simulink model "strain"  (R2024b)
settings: Solver=FixedStepAuto  StartTime=0.0  StopTime=inf  RelTol=1e-3  EnableMultiTasking=on
libraries: fl_lib x5, nesl_utility x4, stm32f4xxblockslib x2, ee_lib x2
settings Model: STM32="{\"AnalogInput\":[{\"ID\":\"untitled1:2\"},{\"ID\":\"strain:206\"}],\"DigitalPortRead\":{\"ID\":\"strain:210\"}}"  Creator=Lenovo  LastModifiedBy=Lenovo
settings OptimizationCC: BlockReduction=off  DefaultParameterBehavior=Inlined  BufferReuse=off  EnhancedBackFolding=on  PassReuseOutputArgsAs=Individual arguments  ZeroExternalMemoryAtStartup=off  ZeroInternalMemoryAtStartup=off  MaxStackSize=512  OptimizeBlockOrder=speed  DifferentSizesBufferReuse=on  EfficientTunableParamExpr=on
settings DebuggingCC: ParameterTunabilityLossMsg=error
settings HardwareCC: ProdBitPerPointer=32  ProdBitPerSizeT=32  ProdBitPerPtrDiffT=32  ProdLargestAtomicInteger=Long  ProdLargestAtomicFloat=Double  ProdWordSize=32  ProdLongLongMode=on  ProdHWDeviceType=ARM Compatible->ARM Cortex-M
settings SFSimCC: MATLABDynamicMemAlloc=off
settings RTWCC: Description=Embedded Coder  SystemTargetFile=ert.tlc  HardwareBoard=STM32G4xx Based  TemplateMakefile=ert_default_tmf  Toolchain=GNU Tools for ARM Embedded Processors
settings CodeAppCC: ForceParamTrailComments=on  IgnoreCustomStorageClasses=off  OperatorAnnotations=on  SimulinkDataObjDesc=on  SFDataObjDesc=on  InsertBlockDesc=on
settings ERTTargetCC: TargetLangStandard=C99 (ISO)  CodeReplacementLibrary=ARM Cortex-M  ExtModeTransport=3  ExtModeStaticAlloc=on  ExtModeStaticAllocSize=2048  ExtModeMexFile=ext_xcp  ExtModeIntrfLevel=Level2 - Open

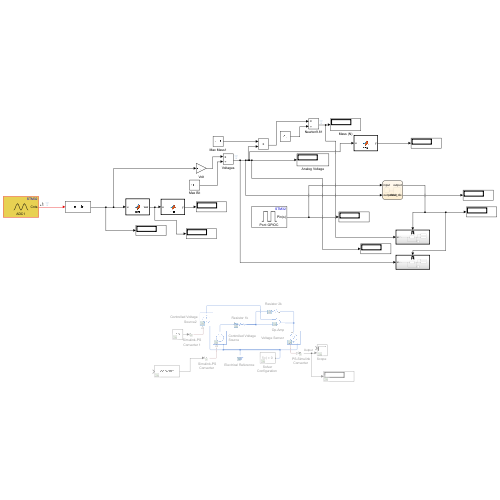
[thumbnail: Simulink's stored preview of the top-level diagram]
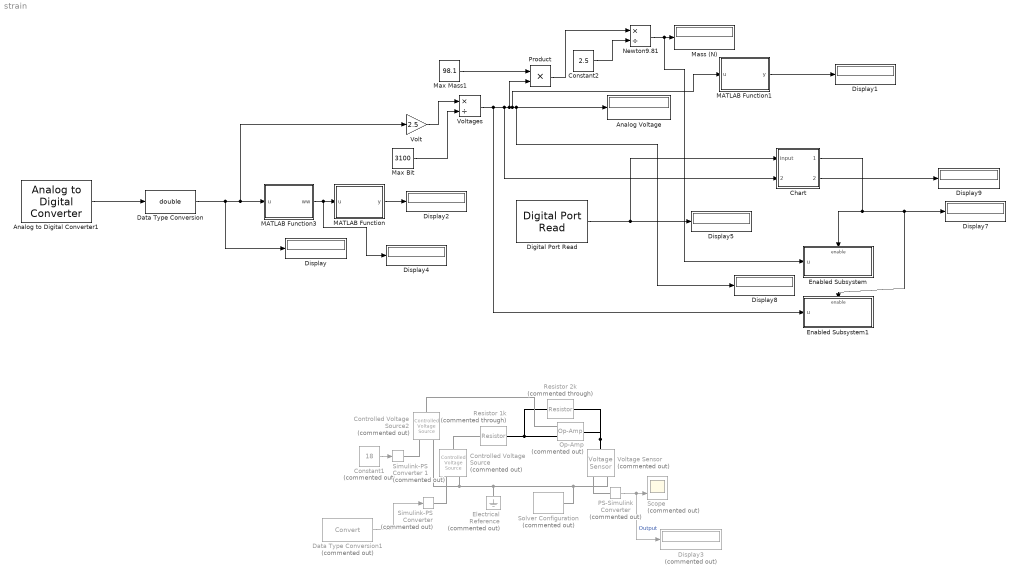
== system strain ==
  Analog Voltage : Display
  Analog to Digital Converter1 : stm32f4xxblockslib/Analog to Digital Converter  ADCModule=ADC1  ConversionGroup=Regular  TriggerMode=Trigger and read  NumberOfConversions=1  EnableBufferConv=off  BufferLength=1  OutputStatus=off  SampleTime=-1  EnableSimPort=off  hoistedMaskSrc=ECSoC/ECSimCodegen/Analog to Digital Converter
  Chart : Stateflow chart  TreatAsAtomicUnit=on
  Constant1 : Constant  Commented=on  Value=18
  Constant2 : Constant  Value=2.5
  "Controlled Voltage Source  " : fl_lib/Electrical/Electrical Sources/Controlled Voltage Source  Commented=on
  "Controlled Voltage Source2 " : fl_lib/Electrical/Electrical Sources/Controlled Voltage Source  Commented=on
  Data Type Conversion : DataTypeConversion  OutDataTypeStr=double  SaturateOnIntegerOverflow=off  RndMeth=Floor
  Data Type Conversion1 : DataTypeConversion  Commented=on  SaturateOnIntegerOverflow=off  RndMeth=Floor
  Digital Port Read : stm32f4xxblockslib/Digital Port Read  PortName=GPIOC  PinNumber=[13]  ReadOperation=on  IOAsArray=on  SampleTime=-1  EnableSimPort=off  hoistedMaskSrc=ECSoC/ECSimCodegen/Digital Port Read
      settings: LibrarySourceBlock=stm32g4xxblockslib/Digital Port Read
  Display{,1..2,4..5,7..9} (8 alike) : Display
      Display2 settings: Format=short_e
  Display3 : Display  Commented=on
  "Electrical Reference " : fl_lib/Electrical/Electrical Elements/Electrical Reference  Commented=on
  Enabled Subsystem : Subsystem  TreatAsAtomicUnit=on
  Enabled Subsystem1 : Subsystem  TreatAsAtomicUnit=on
  MATLAB Function : MATLAB Function  TreatAsAtomicUnit=on
  MATLAB Function1 : MATLAB Function  TreatAsAtomicUnit=on
  MATLAB Function3 : MATLAB Function  TreatAsAtomicUnit=on
  Mass (N) : Display
  Max Bit : Constant  Value=3100
  Max Mass1 : Constant  Value=98.1
  Newton9.81 : Product  Inputs=*/
  "Op-Amp " : fl_lib/Electrical/Electrical Elements/Op-Amp  Commented=on  outI_specify=off  outI_priority=None  outI=0 A  outI_nominal_specify=off  outI_nominal_value=1  outI_nominal_unit=A
  "PS-Simulink Converter " : nesl_utility/PS-Simulink Converter  Commented=on  PhysicalDomain=network_engine_domain  SubClassName=ps_output  LeftPortType=input  RightPortType=output  PseudoPeriodic=off  Frequencies=[]  VectorFormat=inherit  Unit=inherit  AffineConversion=off
  Product : Product
  Resistor 1k : ee_lib/Passive/Resistor  Commented=through  R=1 kOhm  enable_R_tol=0  R_tol=5  tol_distribution=1  nSigma=4  enable_operating_limits=0  operating_limit_action=2  power_rating=1 W  max_working_voltage=100 V  noise_mode=0  Tdevice=25 degC  sample_time=1e-3 s  repeatability=1  user_seed=0  auto_seed=3499211588  fault_action=simscape.enum.assert.action.none  t_fault=1 s  power_derating_T1=70 degC  power_derating_T2=155 degC  operating_temperature_range_vec=[-50, 150] degC  alpha=3.93e-3 1/K  Tmeas=25 degC  thermal_mass=100 J/K  temperature_specify=off  temperature_priority=High  temperature=298.15 K  temperature_nominal_specify=off  temperature_nominal_value=1  temperature_nominal_unit=K
  Resistor 2k : ee_lib/Passive/Resistor  Commented=through  R=2 kOhm  enable_R_tol=ee.enum.toleranceApplication.none  R_tol=5  tol_distribution=1  nSigma=4  enable_operating_limits=ee.enum.enable.no  operating_limit_action=2  power_rating=1 W  max_working_voltage=100 V  noise_mode=0  Tdevice=25 degC  sample_time=1e-3 s  repeatability=1  user_seed=0  auto_seed=3890346746  fault_action=simscape.enum.assert.action.none  t_fault=1 s  power_derating_T1=70 degC  power_derating_T2=155 degC  operating_temperature_range_vec=[-50, 150] degC  alpha=3.93e-3 1/K  Tmeas=25 degC  thermal_mass=100 J/K  temperature_specify=off  temperature_priority=High  temperature=298.15 K  temperature_nominal_specify=off  temperature_nominal_value=1  temperature_nominal_unit=K
  "Scope " : Scope  Commented=on  NumInputPorts=2
  "Simulink-PS Converter " : nesl_utility/Simulink-PS Converter  Commented=on  PhysicalDomain=network_engine_domain  SubClassName=ps_input  LeftPortType=input  RightPortType=output  PseudoPeriodic=off  Frequencies=[]  NoiseDistribution=none  NoiseParameters=[]  Unit=1  AffineConversion=off  FilteringAndDerivatives=provide  SimscapeFilterOrder=1  InputFilterTimeConstant=0.001  UdotUserProvided=0
  Simulink-PS Converter 1 : nesl_utility/Simulink-PS Converter  Commented=on  PhysicalDomain=network_engine_domain  SubClassName=ps_input  LeftPortType=input  RightPortType=output  PseudoPeriodic=off  Frequencies=[]  NoiseDistribution=none  NoiseParameters=[]  Unit=1  AffineConversion=off  FilteringAndDerivatives=provide  SimscapeFilterOrder=1  InputFilterTimeConstant=0.001  UdotUserProvided=0
  "Solver Configuration " : nesl_utility/Solver Configuration  Commented=on  PhysicalDomain=network_engine_domain  SubClassName=solver  LeftPortType=input  RightPortType=generic  Tones=[]  Harmonics=[]  SimulateNoise=off  Profile=off  UseLocalSampling=off  EnableSwitchedLinearOptims=on  FrequencyDomain=off  UseCCode=off  RelTol=0.001  AbsTol=0.001  MinStep=1e-09  ToWorkspace=off  RevertToSquareIcSolve=off  NumHomotopyIterations=100  PhasorMode=off  PhasorModeNumHarmonics=1  ConsistencySolver=NEWTON_FTOL  IndexReductionMethod=DerivativeReplacement  DoDC=off  ResidualTolerance=1e-09  ConsistencyTolSource=GLOBAL  ConsistencyAbsTol=0.001  ConsistencyRelTol=0.001  ConsistencyTolFactor=0.001  UseLocalSolver=off  LocalSolverChoice=NE_BACKWARD_EULER_ADVANCER  ResolveIndetEquations=on  FunctionEvalNumThread=1  LocalSolverSampleTime=0.001  DoFixedCost=off  MaxNonlinIter=3  MaxModeIter=2  ComputeImpulses=off  ImpulseIterations=2  LinearAlgebra=auto  LinearAlgebraNumThread=0  EquationFormulation=NE_TIME_EF  DelaysMemoryBudget=1024  AutomaticFiltering=on  FilteringTimeConstant=0.001  PartitionStorageMethod=AS_NEEDED  PartitionMemoryBudget=1024  PartitionMethod=ROBUST  MultibodyUseLocalSolver=off  MultibodyLocalSolverChoice=ODE1  MultibodyLocalSolverSampleTime=0.001
  Volt : Gain  Gain=2.5
  "Voltage Sensor " : fl_lib/Electrical/Electrical Sensors/Voltage Sensor  Commented=on
  Voltages : Product  Inputs=*/
  wires:
  Constant1/1 -> Simulink-PS Converter 1/1
  "PS-Simulink Converter "/1 -> Display3/1, "Scope "/2  "Output"
  Data Type Conversion1/1 -> "Simulink-PS Converter "/1
  Max Bit/1 -> Voltages/2
  MATLAB Function/1(y) -> Display2/1
  Analog to Digital Converter1/1 -> Data Type Conversion/1
  Newton9.81/1 -> Enabled Subsystem/1(u), Mass (N)/1
  Data Type Conversion/1 -> Volt/1, MATLAB Function3/1(u), Display/1
  Chart/2(time_dis) -> Display9/1
  Constant2/1 -> Newton9.81/2
  Voltages/1 -> Enabled Subsystem1/1(u), Chart/2(outputvolt), Product/2, MATLAB Function1/1(u), Analog Voltage/1, Display8/1
  Chart/1(output) -> Enabled Subsystem1/Enable, Display7/1, Enabled Subsystem/Enable
  MATLAB Function1/1(y) -> Display1/1
  MATLAB Function3/1(ww) -> Display4/1, MATLAB Function/1(u)
  Max Mass1/1 -> Product/1
  Product/1 -> Newton9.81/1
  Digital Port Read/1 -> Chart/1(input), Display5/1
  Volt/1 -> Voltages/1
  connections:
  "Solver Configuration "/RConn1 -- "Electrical Reference "/LConn1 -- "Controlled Voltage Source2 "/RConn2 -- "Controlled Voltage Source  "/RConn2 -- "Voltage Sensor "/RConn2
  Resistor 2k/RConn1 -- "Op-Amp "/LConn2 -- Resistor 1k/RConn1
  "Voltage Sensor "/LConn1 -- "Op-Amp "/RConn1 -- Resistor 2k/LConn1
  "Controlled Voltage Source  "/LConn1 -- Resistor 1k/LConn1
  "Voltage Sensor "/RConn1 -- "PS-Simulink Converter "/LConn1
  "Controlled Voltage Source2 "/LConn1 -- "Op-Amp "/LConn1
  Simulink-PS Converter 1/RConn1 -- "Controlled Voltage Source2 "/RConn1
  "Simulink-PS Converter "/RConn1 -- "Controlled Voltage Source  "/RConn1

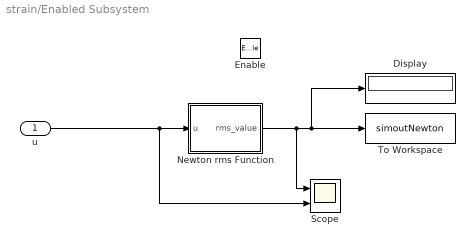
== system strain/Enabled Subsystem ==
  u : Inport
  Enable : EnablePort
  Display : Display
  Newton rms Function : MATLAB Function  TreatAsAtomicUnit=on
  Scope : Scope  NumInputPorts=2
  To Workspace : ToWorkspace  VariableName=simoutNewton  SaveFormat=Timeseries  SampleTime=-1
  wires:
  u/1 -> Scope/2, Newton rms Function/1(u)
  Newton rms Function/1(rms_value) -> Scope/1, Display/1, To Workspace/1

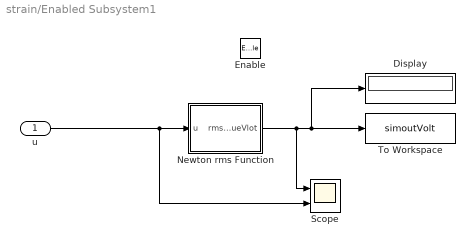
== system strain/Enabled Subsystem1 ==
  u : Inport
  Enable : EnablePort
  Display : Display
  Newton rms Function : MATLAB Function  TreatAsAtomicUnit=on
  Scope : Scope  NumInputPorts=2
  To Workspace : ToWorkspace  VariableName=simoutVolt  SaveFormat=Timeseries  SampleTime=-1
  wires:
  u/1 -> Scope/2, Newton rms Function/1(u)
  Newton rms Function/1(rms_valueVlot) -> Scope/1, Display/1, To Workspace/1

== matlab function strain/MATLAB Function ==
  data: u input; y output
function y = fcn(u)
y = u/0.3;
if y <0
    y=0;
end

== matlab function strain/Enabled Subsystem/Newton rms Function ==
  data: u input; rms_value output
function rms_value = fcn(u)
    % Get the size of input data u
    n = 1;  % Determine how many elements are in u
    
    % Initialize an array to store the 1000 data points
    persistent data_array;  % Use persistent to store data across function calls
    persistent count;       % To keep track of how many data points have been stored
    
    if isempty(data_array)
        data_array = zeros(1000, 1);  % Preallocate space for 1000 data points
        count = 0;                    % Initialize the count
    end
    
    % Loop through each element of the input data and store it
    for i = 1:n
        if count < 1000
            count = count + 1;
            data_array(count) = u(i);  % Store the data
        end
    end
    
    % Once 1000 data points have been stored, calculate the RMS
    if count == 1000
        % Calculate the RMS value
        rms_value = sqrt(mean(data_array.^2));
        
        % Reset the count and data_array if needed for continuous calculations
        count = 0;
        data_array = zeros(1000, 1);
    else
        rms_value = NaN;  % Output NaN until 1000 points have been collected
    end
   
end

== stateflow chart strain/Chart ==
  state initial
    entry:
    time=0;
    outputvolt;
    output= 0;
  state State
    entry:
    output = 1;
    during:
    time = time + 0.001;
    time_dis = time;
    exit:
    output = 0;
    time = 0;
  (default) -> initial
  initial -> State : [input == 1]
  State -> initial : [time >= 1]
  data: input input; outputvolt input; output output; time local; time_dis output

== matlab function strain/MATLAB Function1 ==
  data: u input; y output
function y = fcn(u)
y = u/0.31;
if y <0
    y=0;
end

== matlab function strain/Enabled Subsystem1/Newton rms Function ==
  data: u input; rms_valueVlot output
function rms_valueVlot = fcn(u)
    % Get the size of input data u
    n = 1;  % Determine how many elements are in u
    
    % Initialize an array to store the 1000 data points
    persistent data_array;  % Use persistent to store data across function calls
    persistent count;       % To keep track of how many data points have been stored
    
    if isempty(data_array)
        data_array = zeros(1000, 1);  % Preallocate space for 1000 data points
        count = 0;                    % Initialize the count
    end
    
    % Loop through each element of the input data and store it
    for i = 1:n
        if count < 1000
            count = count + 1;
            data_array(count) = u(i);  % Store the data
        end
    end
    
    % Once 1000 data points have been stored, calculate the RMS
    if count == 1000
        % Calculate the RMS value
        rms_valueVlot = sqrt(mean(data_array.^2));
        
        % Reset the count and data_array if needed for continuous calculations
        count = 0;
        data_array = zeros(1000, 1);
    else
        rms_valueVlot = NaN;  % Output NaN until 1000 points have been collected
    end
   
end

== matlab function strain/MATLAB Function3 ==
  data: u input; ww output
function ww= fcn(u)
ww = u -30;
if(ww < 0)
    ww = 0;
end
